simulink model "SimulationLQR-v2024"  (R2024b)
settings: Solver=VariableStepAuto  StartTime=0.0  StopTime=40  MaxStep=0.01  RelTol=1e-10
undefined symbols (not defined in the file): A, B, C, D, K
settings Model: Creator=Igor  LastModifiedBy=Igor
settings ConfigComp: CovBoundaryAbsTol=1.0e-5

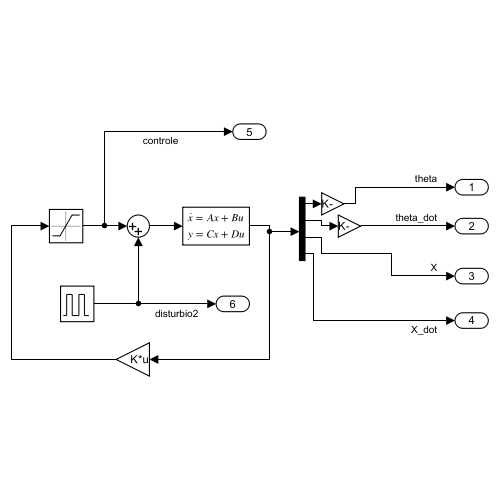
[thumbnail: Simulink's stored preview of the top-level diagram]
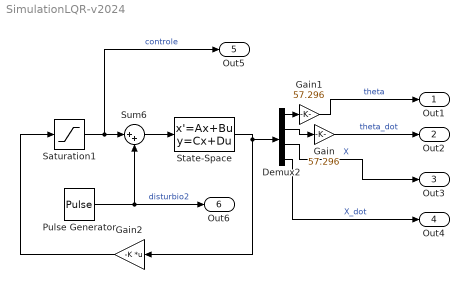
== system SimulationLQR-v2024 ==
  Demux2 : Demux
  Gain : Gain  Gain=57.296
  Gain1 : Gain  Gain=57.296
  Gain2 : Gain  Gain=-K  Multiplication=Matrix(K*u)
  Pulse Generator : DiscretePulseGenerator  PulseType=Time based  Amplitude=3  Period=100  PulseWidth=99  PhaseDelay=1
  Saturation1 : Saturate  UpperLimit=12  LowerLimit=-12
  State-Space : StateSpace  A=A  B=B  C=C  D=D  InitialCondition=0
  Sum6 : Sum  Inputs=|++
  Out1 : Outport
  Out2 : Outport  Port=2
  Out3 : Outport  Port=3
  Out4 : Outport  Port=4
  Out5 : Outport  Port=5
  Out6 : Outport  Port=6
  wires:
  Demux2/3 -> Out3/1  "X"
  State-Space/1 -> Demux2/1, Gain2/1
  Sum6/1 -> State-Space/1
  Saturation1/1 -> Out5/1, Sum6/1  "controle"
  Demux2/1 -> Gain1/1
  Demux2/2 -> Gain/1
  Gain/1 -> Out2/1  "theta_dot"
  Gain1/1 -> Out1/1  "theta"
  Gain2/1 -> Saturation1/1
  Pulse Generator/1 -> Out6/1, Sum6/2  "disturbio2"
  Demux2/4 -> Out4/1  "X_dot"
